simulink model "arm_robot"  (R2020b)
settings: Solver=VariableStepAuto  StartTime=0.0  StopTime=10.0  RelTol=1e-3  AbsTol=1e-3  EnableMultiTasking=on
undefined symbols (not defined in the file): X, Y, Z
libraries: sm_lib x15, nesl_utility x4
settings Model: Creator=何君阔  LastModifiedBy=何君阔
settings SolverCC: AutoScaleAbsTol=off
settings DataIOCC: LimitDataPoints=on  MaxDataPoints=10000
settings OptimizationCC: LifeSpan=inf
settings DebuggingCC: AllowSymbolicDim=off  SFUnexpectedBacktrackingDiag=warning  SFNoUnconditionalDefaultTransitionDiag=warning  SFExecutionAtInitializationDiag=none  ArithmeticOperatorsInVariantConditions=warning
settings SFSimCC: SimUseLocalCustomCode=off  CustomCodeUndefinedFunction=UseInterfaceOnly
settings RTWCC: RTWUseLocalCustomCode=off
settings CodeAppCC: StateflowObjectComments=on
settings GRTTargetCC: TargetLangStandard=C89/C90 (ANSI)
settings ConfigComp: CovMetricSettings=dw  CovSaveCumulativeToWorkspaceVar=on  CovSaveSingleToWorkspaceVar=on  CovExternalEMLEnable=off  CovSFcnEnable=off
settings SimscapeCC: SimscapeLogType=all  SimscapeLogSimulationStatistics=on  SimscapeLogDataHistory=10000

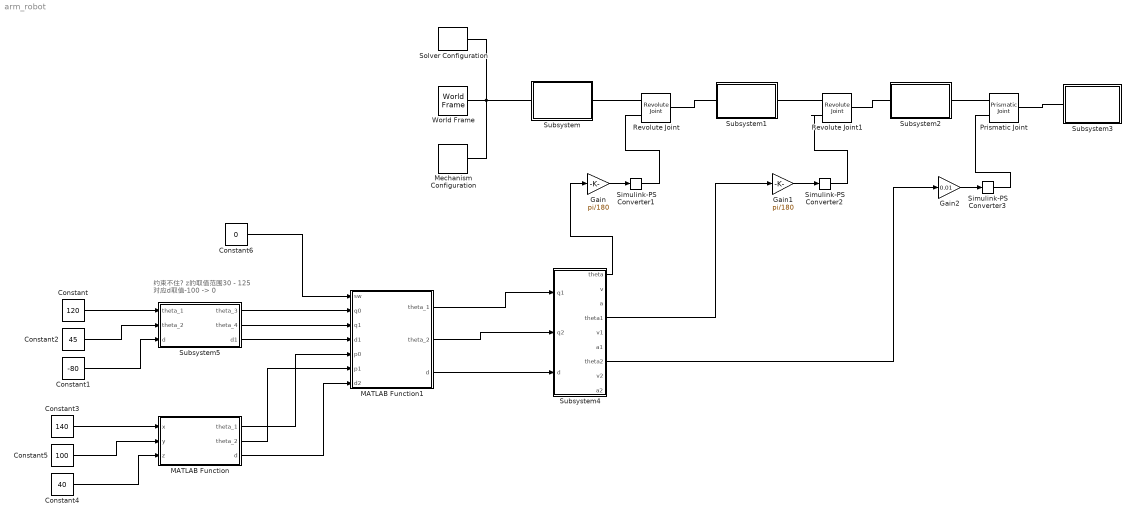
== system arm_robot ==
  note: 约束不住? z的取值范围30 - 125
      | 对应d取值-100 -> 0
  Constant : Constant  Value=120
  Constant1 : Constant  Value=-80
  Constant2 : Constant  Value=45
  Constant3 : Constant  Value=140
  Constant4 : Constant  Value=40
  Constant5 : Constant  Value=100
  Constant6 : Constant  Value=0
  Gain : Gain  Gain=pi/180
  Gain1 : Gain  Gain=pi/180
  Gain2 : Gain  Gain=0.01
  MATLAB Function : MATLAB Function  TreatAsAtomicUnit=on
  MATLAB Function1 : MATLAB Function  TreatAsAtomicUnit=on
  Mechanism Configuration : sm_lib/Utilities/Mechanism Configuration  UniformGravity=Constant  GravityVector=[0 0 -9.80665]  GravityVectorUnits=m/s^2  GravityUnits=m/s^2  LinearizationDelta=0.001  JointModeTransitionNonlinearIterations=2
      settings: SourceProductName=Multibody
  Prismatic Joint : sm_lib/Joints/Prismatic Joint  JointMode=Normal  SenseConstraintForce=off  SenseConstraintForceX=off  SenseConstraintForceY=off  SenseConstraintForceZ=off  SenseConstraintTorque=off  SenseConstraintTorqueX=off  SenseConstraintTorqueY=off  SenseConstraintTorqueZ=off  SenseTotalForce=off  SenseTotalForceX=off  SenseTotalForceY=off  SenseTotalForceZ=off  SenseTotalTorque=off  SenseTotalTorqueX=off  SenseTotalTorqueY=off  SenseTotalTorqueZ=off  CompositeWrenchDir=FollowerOnBase  CompositeWrenchFrame=BaseFrame  EquilibriumPosition=0  EquilibriumPositionUnits=m  SpringStiffness=0  SpringStiffnessUnits=N/m  DampingCoefficient=0  DampingCoefficientUnits=N/(m/s)  TorqueActuationMode=ComputedTorque  MotionActuationMode=InputMotion  SensePosition=off  SenseVelocity=off  SenseAcceleration=off  SenseTorqueForce=off  SenseLowerLimitTorqueForce=off  SenseUpperLimitTorqueForce=off  LowerLimitSpecify=on  LowerLimitBound=-100  LowerLimitBoundUnits=cm  LowerLimitStiffness=1e6  LowerLimitStiffnessUnits=N/m  LowerLimitDamping=1e3  LowerLimitDampingUnits=N/(m/s)  LowerLimitTransitionRegionWidth=1e-4  LowerLimitTransitionRegionWidthUnits=m  UpperLimitSpecify=on  UpperLimitBound=0  UpperLimitBoundUnits=cm  UpperLimitStiffness=1e6  UpperLimitStiffnessUnits=N/m  UpperLimitDamping=1e3  UpperLimitDampingUnits=N/(m/s)  UpperLimitTransitionRegionWidth=1e-4  UpperLimitTransitionRegionWidthUnits=m  PositionTargetSpecify=off  PositionTargetPriority=High  PositionTargetValue=0  PositionTargetValueUnits=m  VelocityTargetSpecify=off  VelocityTargetPriority=High  VelocityTargetValue=0  VelocityTargetValueUnits=m/s
  Revolute Joint : sm_lib/Joints/Revolute Joint  JointMode=Normal  SenseConstraintForce=off  SenseConstraintForceX=off  SenseConstraintForceY=off  SenseConstraintForceZ=off  SenseConstraintTorque=off  SenseConstraintTorqueX=off  SenseConstraintTorqueY=off  SenseConstraintTorqueZ=off  SenseTotalForce=off  SenseTotalForceX=off  SenseTotalForceY=off  SenseTotalForceZ=off  SenseTotalTorque=off  SenseTotalTorqueX=off  SenseTotalTorqueY=off  SenseTotalTorqueZ=off  CompositeWrenchDir=FollowerOnBase  CompositeWrenchFrame=BaseFrame  EquilibriumPosition=0  EquilibriumPositionUnits=deg  SpringStiffness=0  SpringStiffnessUnits=N*m/deg  DampingCoefficient=0  DampingCoefficientUnits=N*m/(deg/s)  TorqueActuationMode=ComputedTorque  MotionActuationMode=InputMotion  SensePosition=off  SenseVelocity=off  SenseAcceleration=off  SenseTorqueForce=off  SenseLowerLimitTorqueForce=off  SenseUpperLimitTorqueForce=off  LowerLimitSpecify=off  LowerLimitBound=-90  LowerLimitBoundUnits=deg  LowerLimitStiffness=1e4  LowerLimitStiffnessUnits=N*m/deg  LowerLimitDamping=10  LowerLimitDampingUnits=N*m/(deg/s)  LowerLimitTransitionRegionWidth=0.1  LowerLimitTransitionRegionWidthUnits=deg  UpperLimitSpecify=off  UpperLimitBound=90  UpperLimitBoundUnits=deg  UpperLimitStiffness=1e4  UpperLimitStiffnessUnits=N*m/deg  UpperLimitDamping=10  UpperLimitDampingUnits=N*m/(deg/s)  UpperLimitTransitionRegionWidth=0.1  UpperLimitTransitionRegionWidthUnits=deg  PositionTargetSpecify=off  PositionTargetPriority=High  PositionTargetValue=0  PositionTargetValueUnits=deg  VelocityTargetSpecify=off  VelocityTargetPriority=High  VelocityTargetValue=0  VelocityTargetValueUnits=deg/s
  Revolute Joint1 : sm_lib/Joints/Revolute Joint  JointMode=Normal  SenseConstraintForce=off  SenseConstraintForceX=off  SenseConstraintForceY=off  SenseConstraintForceZ=off  SenseConstraintTorque=off  SenseConstraintTorqueX=off  SenseConstraintTorqueY=off  SenseConstraintTorqueZ=off  SenseTotalForce=off  SenseTotalForceX=off  SenseTotalForceY=off  SenseTotalForceZ=off  SenseTotalTorque=off  SenseTotalTorqueX=off  SenseTotalTorqueY=off  SenseTotalTorqueZ=off  CompositeWrenchDir=FollowerOnBase  CompositeWrenchFrame=BaseFrame  EquilibriumPosition=0  EquilibriumPositionUnits=deg  SpringStiffness=0  SpringStiffnessUnits=N*m/deg  DampingCoefficient=0  DampingCoefficientUnits=N*m/(deg/s)  TorqueActuationMode=ComputedTorque  MotionActuationMode=InputMotion  SensePosition=off  SenseVelocity=off  SenseAcceleration=off  SenseTorqueForce=off  SenseLowerLimitTorqueForce=off  SenseUpperLimitTorqueForce=off  LowerLimitSpecify=off  LowerLimitBound=-90  LowerLimitBoundUnits=deg  LowerLimitStiffness=1e4  LowerLimitStiffnessUnits=N*m/deg  LowerLimitDamping=10  LowerLimitDampingUnits=N*m/(deg/s)  LowerLimitTransitionRegionWidth=0.1  LowerLimitTransitionRegionWidthUnits=deg  UpperLimitSpecify=off  UpperLimitBound=90  UpperLimitBoundUnits=deg  UpperLimitStiffness=1e4  UpperLimitStiffnessUnits=N*m/deg  UpperLimitDamping=10  UpperLimitDampingUnits=N*m/(deg/s)  UpperLimitTransitionRegionWidth=0.1  UpperLimitTransitionRegionWidthUnits=deg  PositionTargetSpecify=off  PositionTargetPriority=High  PositionTargetValue=0  PositionTargetValueUnits=deg  VelocityTargetSpecify=off  VelocityTargetPriority=High  VelocityTargetValue=0  VelocityTargetValueUnits=deg/s
  Simulink-PS Converter1 : nesl_utility/Simulink-PS Converter  PhysicalDomain=network_engine_domain  SubClassName=ps_input  LeftPortType=input  RightPortType=output  PseudoPeriodic=off  Frequencies=[]  NoiseDistribution=none  NoiseParameters=[]  Unit=rad  AffineConversion=off  FilteringAndDerivatives=filter  SimscapeFilterOrder=2  InputFilterTimeConstant=0.001  UdotUserProvided=0
      settings: SourceProductName=Utilities
  Simulink-PS Converter2 : nesl_utility/Simulink-PS Converter  PhysicalDomain=network_engine_domain  SubClassName=ps_input  LeftPortType=input  RightPortType=output  PseudoPeriodic=off  Frequencies=[]  NoiseDistribution=none  NoiseParameters=[]  Unit=rad  AffineConversion=off  FilteringAndDerivatives=filter  SimscapeFilterOrder=2  InputFilterTimeConstant=0.001  UdotUserProvided=0
      settings: SourceProductName=Utilities
  Simulink-PS Converter3 : nesl_utility/Simulink-PS Converter  PhysicalDomain=network_engine_domain  SubClassName=ps_input  LeftPortType=input  RightPortType=output  PseudoPeriodic=off  Frequencies=[]  NoiseDistribution=none  NoiseParameters=[]  Unit=m  AffineConversion=off  FilteringAndDerivatives=filter  SimscapeFilterOrder=2  InputFilterTimeConstant=0.001  UdotUserProvided=0
      settings: SourceProductName=Utilities
  Solver Configuration : nesl_utility/Solver Configuration  PhysicalDomain=network_engine_domain  SubClassName=solver  LeftPortType=input  RightPortType=generic  Tones=[]  Harmonics=[]  SimulateNoise=off  Profile=off  UseLocalSampling=off  EnableSwitchedLinearOptims=on  FrequencyDomain=off  UseCCode=off  RelTol=0.001  AbsTol=1e-06  MinStep=1e-09  ToWorkspace=off  RevertToSquareIcSolve=off  NumHomotopyIterations=100  PhasorMode=off  PhasorModeNumHarmonics=1  DoDC=off  ResidualTolerance=1e-09  UseLocalSolver=off  LocalSolverChoice=NE_BACKWARD_EULER_ADVANCER  LocalSolverSampleTime=0.001  DoFixedCost=off  MaxNonlinIter=3  MaxModeIter=2  ComputeImpulses=off  ImpulseIterations=2  LinearAlgebra=Sparse  EquationFormulation=NE_TIME_EF  DelaysMemoryBudget=1024  AutomaticFiltering=on  FilteringTimeConstant=0.001  PartitionStorageMethod=AS_NEEDED  PartitionMemoryBudget=1024  PartitionMethod=FAST
      settings: SourceProductName=Utilities
  Subsystem : Subsystem
  Subsystem1 : Subsystem
  Subsystem2 : Subsystem
  Subsystem3 : Subsystem
  Subsystem4 : Subsystem
  Subsystem5 : Subsystem
  World Frame : sm_lib/Frames and Transforms/World Frame
      settings: SourceProductName=Multibody
  wires:
  Gain/1 -> Simulink-PS Converter1/1
  Gain1/1 -> Simulink-PS Converter2/1
  Gain2/1 -> Simulink-PS Converter3/1
  Subsystem4/1(theta) -> Gain/1
  Subsystem4/4(theta1) -> Gain1/1
  Subsystem4/7(theta2) -> Gain2/1
  Constant/1 -> Subsystem5/1(theta_1)
  Constant2/1 -> Subsystem5/2(theta_2)
  Constant1/1 -> Subsystem5/3(d)
  Constant3/1 -> MATLAB Function/1(x)
  Constant5/1 -> MATLAB Function/2(y)
  Constant4/1 -> MATLAB Function/3(z)
  Subsystem5/1(theta_3) -> MATLAB Function1/2(q0)
  Subsystem5/2(theta_4) -> MATLAB Function1/3(q1)
  Subsystem5/3(d1) -> MATLAB Function1/4(d1)
  MATLAB Function/1(theta_1) -> MATLAB Function1/5(p0)
  MATLAB Function/2(theta_2) -> MATLAB Function1/6(p1)
  MATLAB Function/3(d) -> MATLAB Function1/7(d2)
  MATLAB Function1/1(theta_1) -> Subsystem4/1(q1)
  MATLAB Function1/2(theta_2) -> Subsystem4/2(q2)
  MATLAB Function1/3(d) -> Subsystem4/3(d)
  Constant6/1 -> MATLAB Function1/1(sw)
  connections:
  Mechanism Configuration/RConn1 -- Subsystem/LConn1 -- Solver Configuration/RConn1 -- World Frame/RConn1
  Subsystem/RConn1 -- Revolute Joint/LConn1
  Subsystem1/LConn1 -- Revolute Joint/RConn1
  Simulink-PS Converter1/RConn1 -- Revolute Joint/LConn2
  Subsystem1/RConn1 -- Revolute Joint1/LConn1
  Revolute Joint1/RConn1 -- Subsystem2/LConn1
  Revolute Joint1/LConn2 -- Simulink-PS Converter2/RConn1
  Prismatic Joint/LConn1 -- Subsystem2/RConn1
  Simulink-PS Converter3/RConn1 -- Prismatic Joint/LConn2
  Subsystem3/LConn1 -- Prismatic Joint/RConn1

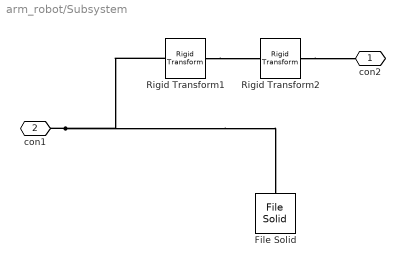
== system arm_robot/Subsystem ==
  File Solid : sm_lib/Body Elements/File Solid  ExtGeomFileName=E:\robot_work\基座 v1.step  UnitType=Custom  ExtGeomFileUnits=mm  StepReaderType=HEX  ExportConvexHullGeometry=off  InertiaType=CalculateFromGeometry  Mass=1  MassUnits=kg  CenterOfMass=[0 0 0]  CenterOfMassUnits=m  MomentsOfInertia=[1 1 1]  MomentsOfInertiaUnits=kg*m^2  ProductsOfInertia=[0 0 0]  ProductsOfInertiaUnits=kg*m^2  BasedOnType=Mass  Density=1000  DensityUnits=kg/m^3  DoExposeReferenceFrame=on  SerializedFrames=<Frames/>  GraphicType=FromGeometry  MarkerShape=Sphere  MarkerSize=10  GraphicVisPropType=SimpleVisualProperties  GraphicDiffuseColor=[0.5 0.5 0.5]  GraphicSpecularColor=[0.5 0.5 0.5 1.0]  GraphicAmbientColor=[0.15 0.15 0.15 1.0]  GraphicEmissiveColor=[0.0 0.0 0.0 1.0]  GraphicShininess=75  GraphicOpacity=1.0
  Rigid Transform1 : sm_lib/Frames and Transforms/Rigid Transform  TranslationMethod=StandardAxis  TranslationStandardOffset=400  TranslationLengthUnit=mm  TranslationStandardAxis=+X  TranslationCartesianOffset=[0 0 0]  TranslationROffset=0  TranslationROffsetUnits=m  TranslationZOffset=0  TranslationZOffsetUnits=m  TranslationThetaOffset=0  TranslationThetaOffsetUnits=deg  RotationMethod=None  RotationAngleUnits=deg  RotationStandardAxis=+Z  RotationAngle=0.0  RotationArbitraryAxis=[0 0 1]  FollAlignAxisA=+X  BaseAlignAxisA=+Y  FollAlignAxisB=+Y  BaseAlignAxisB=+Z  RotationSequenceAxes=FollowerAxes  RotationSequence=XYX  RotationSequenceAngles=[0 0 0]  RotationSequenceAnglesUnits=deg  RotationMatrix=[1 0 0; 0 1 0; 0 0 1]
      settings: SourceProductName=Multibody
  Rigid Transform2 : sm_lib/Frames and Transforms/Rigid Transform  TranslationMethod=StandardAxis  TranslationStandardOffset=150  TranslationLengthUnit=cm  TranslationStandardAxis=+Z  TranslationCartesianOffset=[0 0 0]  TranslationROffset=0  TranslationROffsetUnits=m  TranslationZOffset=0  TranslationZOffsetUnits=m  TranslationThetaOffset=0  TranslationThetaOffsetUnits=deg  RotationMethod=None  RotationAngleUnits=deg  RotationStandardAxis=+Z  RotationAngle=0.0  RotationArbitraryAxis=[0 0 1]  FollAlignAxisA=+X  BaseAlignAxisA=+Y  FollAlignAxisB=+Y  BaseAlignAxisB=+Z  RotationSequenceAxes=FollowerAxes  RotationSequence=XYX  RotationSequenceAngles=[0 0 0]  RotationSequenceAnglesUnits=deg  RotationMatrix=[1 0 0; 0 1 0; 0 0 1]
      settings: SourceProductName=Multibody
  con2 : PMIOPort  Side=Right
  con1 : PMIOPort  Port=2  Side=Left
  connections:
  con1/RConn1 -- File Solid/RConn1 -- Rigid Transform1/LConn1
  Rigid Transform1/RConn1 -- Rigid Transform2/LConn1
  Rigid Transform2/RConn1 -- con2/RConn1

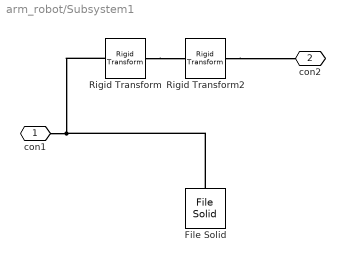
== system arm_robot/Subsystem1 ==
  File Solid : sm_lib/Body Elements/File Solid  ExtGeomFileName=E:\robot_work\link_1.step  UnitType=Custom  ExtGeomFileUnits=mm  StepReaderType=HEX  ExportConvexHullGeometry=off  InertiaType=CalculateFromGeometry  Mass=1  MassUnits=kg  CenterOfMass=[0 0 0]  CenterOfMassUnits=m  MomentsOfInertia=[1 1 1]  MomentsOfInertiaUnits=kg*m^2  ProductsOfInertia=[0 0 0]  ProductsOfInertiaUnits=kg*m^2  BasedOnType=Mass  Density=1000  DensityUnits=kg/m^3  DoExposeReferenceFrame=on  SerializedFrames=<Frames/>  GraphicType=FromGeometry  MarkerShape=Sphere  MarkerSize=10  GraphicVisPropType=SimpleVisualProperties  GraphicDiffuseColor=[0.5 0.5 0.5]  GraphicSpecularColor=[0.5 0.5 0.5 1.0]  GraphicAmbientColor=[0.15 0.15 0.15 1.0]  GraphicEmissiveColor=[0.0 0.0 0.0 1.0]  GraphicShininess=75  GraphicOpacity=1.0
  Rigid Transform : sm_lib/Frames and Transforms/Rigid Transform  TranslationMethod=StandardAxis  TranslationStandardOffset=100  TranslationLengthUnit=cm  TranslationStandardAxis=+X  TranslationCartesianOffset=[0 0 0]  TranslationROffset=0  TranslationROffsetUnits=m  TranslationZOffset=0  TranslationZOffsetUnits=m  TranslationThetaOffset=0  TranslationThetaOffsetUnits=deg  RotationMethod=None  RotationAngleUnits=deg  RotationStandardAxis=-Y  RotationAngle=90  RotationArbitraryAxis=[0 0 1]  FollAlignAxisA=+X  BaseAlignAxisA=+Y  FollAlignAxisB=+Y  BaseAlignAxisB=+Z  RotationSequenceAxes=FollowerAxes  RotationSequence=XYX  RotationSequenceAngles=[0 0 0]  RotationSequenceAnglesUnits=deg  RotationMatrix=[1 0 0; 0 1 0; 0 0 1]
      settings: SourceProductName=Multibody
  Rigid Transform2 : sm_lib/Frames and Transforms/Rigid Transform  TranslationMethod=StandardAxis  TranslationStandardOffset=30  TranslationLengthUnit=cm  TranslationStandardAxis=+Z  TranslationCartesianOffset=[0 0 0]  TranslationROffset=0  TranslationROffsetUnits=m  TranslationZOffset=0  TranslationZOffsetUnits=m  TranslationThetaOffset=0  TranslationThetaOffsetUnits=deg  RotationMethod=None  RotationAngleUnits=deg  RotationStandardAxis=+Y  RotationAngle=90  RotationArbitraryAxis=[0 0 1]  FollAlignAxisA=+X  BaseAlignAxisA=+Y  FollAlignAxisB=+Y  BaseAlignAxisB=+Z  RotationSequenceAxes=FollowerAxes  RotationSequence=XYX  RotationSequenceAngles=[0 0 0]  RotationSequenceAnglesUnits=deg  RotationMatrix=[1 0 0; 0 1 0; 0 0 1]
      settings: SourceProductName=Multibody
  con1 : PMIOPort  Side=Left
  con2 : PMIOPort  Port=2  Side=Right
  connections:
  con1/RConn1 -- File Solid/RConn1 -- Rigid Transform/LConn1
  Rigid Transform/RConn1 -- Rigid Transform2/LConn1
  Rigid Transform2/RConn1 -- con2/RConn1

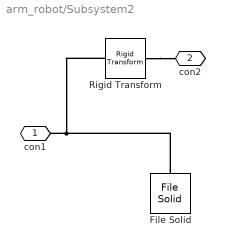
== system arm_robot/Subsystem2 ==
  File Solid : sm_lib/Body Elements/File Solid  ExtGeomFileName=E:\robot_work\link2 v1.step  UnitType=Custom  ExtGeomFileUnits=mm  StepReaderType=HEX  ExportConvexHullGeometry=off  InertiaType=CalculateFromGeometry  Mass=1  MassUnits=kg  CenterOfMass=[0 0 0]  CenterOfMassUnits=m  MomentsOfInertia=[1 1 1]  MomentsOfInertiaUnits=kg*m^2  ProductsOfInertia=[0 0 0]  ProductsOfInertiaUnits=kg*m^2  BasedOnType=Mass  Density=1000  DensityUnits=kg/m^3  DoExposeReferenceFrame=on  SerializedFrames=<Frames/>  GraphicType=FromGeometry  MarkerShape=Sphere  MarkerSize=10  GraphicVisPropType=SimpleVisualProperties  GraphicDiffuseColor=[0.5 0.5 0.5]  GraphicSpecularColor=[0.5 0.5 0.5 1.0]  GraphicAmbientColor=[0.15 0.15 0.15 1.0]  GraphicEmissiveColor=[0.0 0.0 0.0 1.0]  GraphicShininess=75  GraphicOpacity=1.0
  Rigid Transform : sm_lib/Frames and Transforms/Rigid Transform  TranslationMethod=StandardAxis  TranslationStandardOffset=80  TranslationLengthUnit=cm  TranslationStandardAxis=+X  TranslationCartesianOffset=[0 0 0]  TranslationROffset=0  TranslationROffsetUnits=m  TranslationZOffset=0  TranslationZOffsetUnits=m  TranslationThetaOffset=0  TranslationThetaOffsetUnits=deg  RotationMethod=None  RotationAngleUnits=deg  RotationStandardAxis=-Y  RotationAngle=90  RotationArbitraryAxis=[0 0 1]  FollAlignAxisA=+X  BaseAlignAxisA=+Y  FollAlignAxisB=+Y  BaseAlignAxisB=+Z  RotationSequenceAxes=FollowerAxes  RotationSequence=XYX  RotationSequenceAngles=[0 0 0]  RotationSequenceAnglesUnits=deg  RotationMatrix=[1 0 0; 0 1 0; 0 0 1]
      settings: SourceProductName=Multibody
  con1 : PMIOPort  Side=Left
  con2 : PMIOPort  Port=2  Side=Right
  connections:
  Rigid Transform/LConn1 -- File Solid/RConn1 -- con1/RConn1
  Rigid Transform/RConn1 -- con2/RConn1

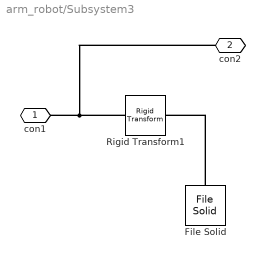
== system arm_robot/Subsystem3 ==
  File Solid : sm_lib/Body Elements/File Solid  ExtGeomFileName=E:\robot_work\link_3.step  UnitType=Custom  ExtGeomFileUnits=mm  StepReaderType=HEX  ExportConvexHullGeometry=off  InertiaType=CalculateFromGeometry  Mass=1  MassUnits=kg  CenterOfMass=[0 0 0]  CenterOfMassUnits=m  MomentsOfInertia=[1 1 1]  MomentsOfInertiaUnits=kg*m^2  ProductsOfInertia=[0 0 0]  ProductsOfInertiaUnits=kg*m^2  BasedOnType=Mass  Density=1000  DensityUnits=kg/m^3  DoExposeReferenceFrame=on  SerializedFrames=<Frames/>  GraphicType=FromGeometry  MarkerShape=Sphere  MarkerSize=10  GraphicVisPropType=SimpleVisualProperties  GraphicDiffuseColor=[0.5 0.5 0.5]  GraphicSpecularColor=[0.5 0.5 0.5 1.0]  GraphicAmbientColor=[0.15 0.15 0.15 1.0]  GraphicEmissiveColor=[0.0 0.0 0.0 1.0]  GraphicShininess=75  GraphicOpacity=1.0
  Rigid Transform1 : sm_lib/Frames and Transforms/Rigid Transform  TranslationMethod=StandardAxis  TranslationStandardOffset=100  TranslationLengthUnit=cm  TranslationStandardAxis=+Z  TranslationCartesianOffset=[0 0 0]  TranslationROffset=0  TranslationROffsetUnits=m  TranslationZOffset=0  TranslationZOffsetUnits=m  TranslationThetaOffset=0  TranslationThetaOffsetUnits=deg  RotationMethod=None  RotationAngleUnits=deg  RotationStandardAxis=+Y  RotationAngle=90  RotationArbitraryAxis=[0 0 1]  FollAlignAxisA=+X  BaseAlignAxisA=+Y  FollAlignAxisB=+Y  BaseAlignAxisB=+Z  RotationSequenceAxes=FollowerAxes  RotationSequence=XYX  RotationSequenceAngles=[0 0 0]  RotationSequenceAnglesUnits=deg  RotationMatrix=[1 0 0; 0 1 0; 0 0 1]
      settings: SourceProductName=Multibody
  con1 : PMIOPort  Side=Left
  con2 : PMIOPort  Port=2  Side=Right
  connections:
  Rigid Transform1/LConn1 -- con2/RConn1 -- con1/RConn1
  File Solid/RConn1 -- Rigid Transform1/RConn1

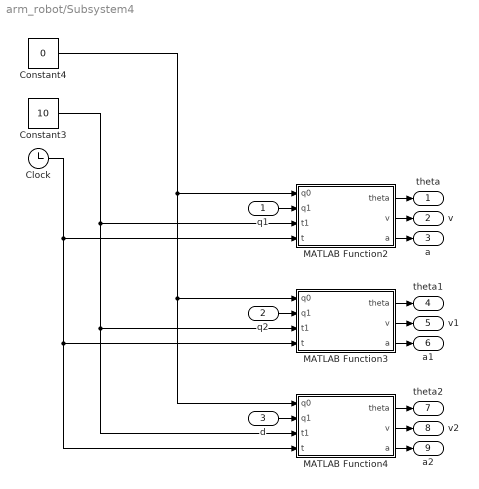
== system arm_robot/Subsystem4 ==
  q1 : Inport
  q2 : Inport  Port=2
  d : Inport  Port=3
  Clock : Clock
  Constant3 : Constant  Value=10
  Constant4 : Constant  Value=0
  MATLAB Function2 : MATLAB Function  TreatAsAtomicUnit=on
  MATLAB Function3 : MATLAB Function  TreatAsAtomicUnit=on
  MATLAB Function4 : MATLAB Function  TreatAsAtomicUnit=on
  theta : Outport
  v : Outport  Port=2
  a : Outport  Port=3
  theta1 : Outport  Port=4
  v1 : Outport  Port=5
  a1 : Outport  Port=6
  theta2 : Outport  Port=7
  v2 : Outport  Port=8
  a2 : Outport  Port=9
  wires:
  Constant3/1 -> MATLAB Function4/3(t1), MATLAB Function3/3(t1), MATLAB Function2/3(t1)
  MATLAB Function2/3(a) -> a/1
  Constant4/1 -> MATLAB Function4/1(q0), MATLAB Function3/1(q0), MATLAB Function2/1(q0)
  MATLAB Function4/2(v) -> v2/1
  MATLAB Function3/2(v) -> v1/1
  q1/1 -> MATLAB Function2/2(q1)
  q2/1 -> MATLAB Function3/2(q1)
  MATLAB Function2/2(v) -> v/1
  Clock/1 -> MATLAB Function4/4(t), MATLAB Function3/4(t), MATLAB Function2/4(t)
  MATLAB Function2/1(theta) -> theta/1
  MATLAB Function4/1(theta) -> theta2/1
  MATLAB Function3/1(theta) -> theta1/1
  MATLAB Function3/3(a) -> a1/1
  d/1 -> MATLAB Function4/2(q1)
  MATLAB Function4/3(a) -> a2/1

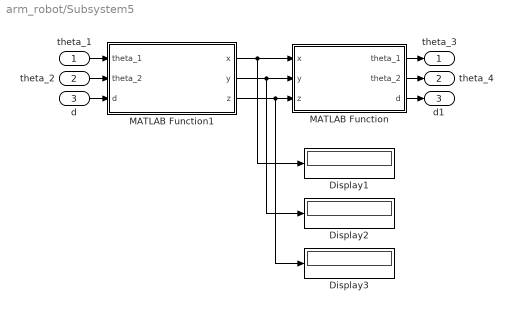
== system arm_robot/Subsystem5 ==
  theta_1 : Inport
  theta_2 : Inport  Port=2
  d : Inport  Port=3
  Display1 : Display
  Display2 : Display
  Display3 : Display
  MATLAB Function : MATLAB Function  TreatAsAtomicUnit=on
  MATLAB Function1 : MATLAB Function  TreatAsAtomicUnit=on
  theta_3 : Outport
  theta_4 : Outport  Port=2
  d1 : Outport  Port=3
  wires:
  MATLAB Function1/3(z) -> Display3/1, MATLAB Function/3(z)
  MATLAB Function1/1(x) -> Display1/1, MATLAB Function/1(x)
  MATLAB Function1/2(y) -> Display2/1, MATLAB Function/2(y)
  d/1 -> MATLAB Function1/3(d)
  MATLAB Function/3(d) -> d1/1
  theta_1/1 -> MATLAB Function1/1(theta_1)
  MATLAB Function/2(theta_2) -> theta_4/1
  theta_2/1 -> MATLAB Function1/2(theta_2)
  MATLAB Function/1(theta_1) -> theta_3/1

== matlab function arm_robot/Subsystem5/MATLAB Function1 ==
  data: x output; theta_1 input; y output; theta_2 input; d input; z output
function [x,y,z] = kinematic_forward(theta_1,theta_2,d)
    L1 = 150;
    L2 = 100;
    L3 = 80;
    x = L2*cos(deg2rad(theta_1))+L3*cos(deg2rad(theta_1+theta_2));
    y = L2*sin(deg2rad(theta_1))+L3*sin(deg2rad(theta_1+theta_2));
    z = L1 - 35 + d;
end

== matlab function arm_robot/Subsystem5/MATLAB Function ==
  data: x input; theta_1 output; y input; z input; theta_2 output; d output
function [theta_1,theta_2,d] = kinematic_inverse(x,y,z)
    L1 = 150;
    L2 = 100;
    L3 = 80;
    if x^2+y^2 > (L1+L2)^2
        error('unreachable point');% 超出工作空间
    end
    d = z - L1 + 35;
    theta_2 = acos((x^2+y^2-L2^2-L3^2)/(2*L2*L3));
    beta = atan2(y,x);
    fai = acos((x^2+y^2+L2^2-L3^2)/(2*L2*sqrt(x^2+y^2)));
    if theta_2 > 0
        theta_1 = beta - fai;
    else
        theta_1 = beta + fai;
    end
    theta_1 = rad2deg(theta_1);
    theta_2 = rad2deg(theta_2);
end

== matlab function arm_robot/Subsystem4/MATLAB Function2 ==
  data: q0 input; theta output; q1 input; t1 input; t input; v output; a output
function [theta,v,a]= Track(q0,q1,t1 ,t)
    a0=q0;
    a1=0;
    v0=0; %起点速度
    v1=0; %终点速度
    a2=(3/(t1)^2)*(q1-q0)-(1/t1)*(2*v0+v1);% 计算三次项参数
    a3=(2/(t1)^3)*(q0-q1)+(1/t1^2)*(v0+v1);

    theta=a0+a1*t+a2*t^2+a3*t^3;% 角度/位移

    v=a1+2*a2*t+3*a3*t^2;% 速度

    a=2*a2+6*a3*t;% 加速度
end

== matlab function arm_robot/Subsystem4/MATLAB Function3 ==
  data: q0 input; theta output; q1 input; t1 input; t input; v output; a output
function [theta,v,a]= Track(q0,q1,t1 ,t)
a0=q0;
a1=0;
v0=0;
v1=0;
a2=(3/(t1)^2)*(q1-q0)-(1/t1)*(2*v0+v1);
a3=(2/(t1)^3)*(q0-q1)+(1/t1^2)*(v0+v1);%计算三次多项式系数

theta=a0+a1*t+a2*t.^2+a3*t.^3;
%v=diff(theta,t);
v=a1+2*a2*t+3*a3*t.^2;
%a=diff(v,t);
a=2*a2+6*a3*t;


%q0=a0;
%q1=a0+a1*t1+a2*t1.^2+a3*.t1.^3;
%v0=a1=0;
%v1=2*a2*t1+3*a3*t1.^2=0;

== matlab function arm_robot/Subsystem4/MATLAB Function4 ==
  data: q0 input; theta output; q1 input; t1 input; t input; v output; a output
function [theta,v,a]= Track(q0,q1,t1 ,t)
a0=q0;
a1=0;
v0=0;
v1=0;
a2=(3/(t1)^2)*(q1-q0)-(1/t1)*(2*v0+v1);
a3=(2/(t1)^3)*(q0-q1)+(1/t1^2)*(v0+v1);%计算三次多项式系数

theta=a0+a1*t+a2*t.^2+a3*t.^3;
%v=diff(theta,t);
v=a1+2*a2*t+3*a3*t.^2;
%a=diff(v,t);
a=2*a2+6*a3*t;


%q0=a0;
%q1=a0+a1*t1+a2*t1.^2+a3*.t1.^3;
%v0=a1=0;
%v1=2*a2*t1+3*a3*t1.^2=0;

== matlab function arm_robot/MATLAB Function ==
  data: x input; theta_1 output; y input; z input; theta_2 output; d output
function [theta_1,theta_2,d] = kinematic_inverse(x,y,z)
    L1 = 150;
    L2 = 100;
    L3 = 80;
    if x^2+y^2 > (L1+L2)^2
        error('unreachable point');% 超出工作空间
    end
    d = z - L1 + 35;
    theta_2 = acos((x^2+y^2-L2^2-L3^2)/(2*L2*L3));
    beta = atan2(y,x);
    fai = acos((x^2+y^2+L2^2-L3^2)/(2*L2*sqrt(x^2+y^2)));
    if theta_2 > 0
        theta_1 = beta - fai;
    else
        theta_1 = beta + fai;
    end
    theta_1 = rad2deg(theta_1);
    theta_2 = rad2deg(theta_2);
end

== matlab function arm_robot/MATLAB Function1 ==
  data: sw input; theta_1 output; q0 input; q1 input; d1 input; p0 input; p1 input; d2 input; theta_2 output; d output
function [theta_1,theta_2,d] = signal_choose(sw,q0,q1,d1,p0,p1,d2)
    if sw == 0
        theta_1 = q0;
        theta_2 = q1;
        d = d1;
    else
        theta_1 = p0;
        theta_2 = p1;
        d = d2;
    end
end
